simulink model "Ex9_5model"  (R2013a)
settings: Solver=ode45  StartTime=0.0  StopTime=5  RelTol=1e5
settings Model: Creator=JLS  LastModifiedBy=John
settings DataIOCC: SignalLoggingSaveFormat=ModelDataLogs
settings OptimizationCC: ExpressionDepthLimit=2147483647
settings DebuggingCC: FcnCallInpInsideContextMsg=UseLocalSettings
settings GRTTargetCC: CombineOutputUpdateFcns=off  GRTInterface=on

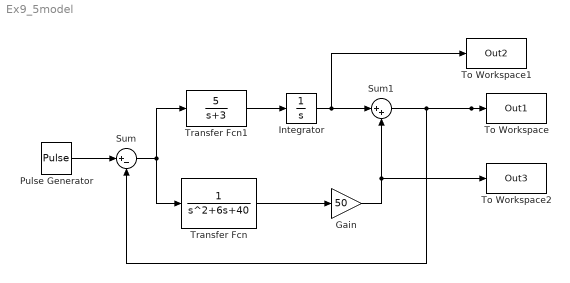
== system Ex9_5model ==
  Gain : Gain  Gain=50
  Integrator : Integrator
  Pulse Generator : DiscretePulseGenerator  PulseType=Time based  Period=10  PulseWidth=5
  Sum : Sum  Inputs=|+-
  Sum1 : Sum  Inputs=|++
  To Workspace : ToWorkspace  VariableName=Out1  SampleTime=-1
  To Workspace1 : ToWorkspace  VariableName=Out2  SampleTime=-1
  To Workspace2 : ToWorkspace  VariableName=Out3  SampleTime=-1
  Transfer Fcn : TransferFcn  Denominator=[1 6 40]
  Transfer Fcn1 : TransferFcn  Numerator=[5]  Denominator=[1 3]
  wires:
  Transfer Fcn1/1 -> Integrator/1
  Integrator/1 -> Sum1/1, To Workspace1/1
  Sum1/1 -> To Workspace/1, Sum/2
  Transfer Fcn/1 -> Gain/1
  Sum/1 -> Transfer Fcn1/1, Transfer Fcn/1
  Gain/1 -> Sum1/2, To Workspace2/1
  Pulse Generator/1 -> Sum/1
